simulink model "Combined_Experiment_Jan23_2020a_NoArm"  (R2020a)
settings: Solver=FixedStepAuto  StartTime=0.0  StopTime=tsim  FixedStep=baseRate  RelTol=1e-3  EnableMultiTasking=on
undefined symbols (not defined in the file): b0, b1, b_out, baseRate, CHASER_ABSOLUTE_POSITION, DiscIntNeverNeededParam, drop_states_ARM, drop_states_BLACK, drop_states_BLUE, drop_states_RED, F_Black_X_nominal, F_Black_Y_nominal, F_Blue_X_nominal, F_Blue_Y_nominal, F_red_X_nominal, F_red_Y_nominal, F_thrusters_BLACK, F_thrusters_BLUE, F_thrusters_RED, Gamma1_el, Gamma1_sh, Gamma1_wr, Gamma2_el, Gamma2_sh, Gamma2_wr, Gamma3_el, Gamma3_sh, Gamma3_wr, Gamma4_el, Gamma4_sh, Gamma4_wr, Gamma5_el, Gamma5_sh, Gamma5_wr, Gamma6_el, Gamma6_sh, Gamma6_wr, HOLD_POINT_RADIUS, home_states_BLACK, home_states_BLUE, home_states_RED, init_states_BLACK, init_states_BLUE, init_states_RED, Kd_tb, Kd_tblue, Kd_tr, Kd_xb, Kd_xblue, Kd_xr, Kd_yb, Kd_yblue, Kd_yr, Kp_tb, Kp_tblue, Kp_tr, Kp_xb, Kp_xblue, Kp_xr, Kp_yb ... (+31)
libraries: dspstat3 x18, raspberrypiBasiclib x10, dspsigops x9, embdlinuxlib x7, MainLibrary x7, simulink x7, mspfiltlib x3, dsparch4 x3, etargetslib x1, sensehatlib x1
(part 9 of 10)

== system Combined_Experiment_Jan23_2020a_NoArm/Phase #3: Experiment/Change BLACK Behavior/Sub-Phase #3 /Custom Discrete PD (Attitude)/x_dot -> x1/Hold this value ==
  In1 : Inport
  Action Port : ActionPort  ActionPortLabel=if(u1 ~= 0)
  Out1 : Outport  VectorParamsAs1DForOutWhenUnconnected=off
  wires:
  In1/1 -> Out1/1

== system Combined_Experiment_Jan23_2020a_NoArm/Phase #3: Experiment/Change BLACK Behavior/Sub-Phase #3 /Custom Discrete PD (X-Position)/x_dot -> x1/Hold this value ==
  In1 : Inport
  Action Port : ActionPort  ActionPortLabel=if(u1 ~= 0)
  Out1 : Outport  VectorParamsAs1DForOutWhenUnconnected=off
  wires:
  In1/1 -> Out1/1

== system Combined_Experiment_Jan23_2020a_NoArm/Phase #3: Experiment/Change BLACK Behavior/Sub-Phase #3 /Custom Discrete PD (Y-Position)/x_dot -> x1/Hold this value ==
  In1 : Inport
  Action Port : ActionPort  ActionPortLabel=if(u1 ~= 0)
  Out1 : Outport  VectorParamsAs1DForOutWhenUnconnected=off
  wires:
  In1/1 -> Out1/1

== system Combined_Experiment_Jan23_2020a_NoArm/Phase #3: Experiment/Change BLACK Behavior/Sub-Phase #4/Custom Discrete PD (Attitude)/x_dot -> x1/Hold this value ==
  In1 : Inport
  Action Port : ActionPort  ActionPortLabel=if(u1 ~= 0)
  Out1 : Outport  VectorParamsAs1DForOutWhenUnconnected=off
  wires:
  In1/1 -> Out1/1

== system Combined_Experiment_Jan23_2020a_NoArm/Phase #3: Experiment/Change BLACK Behavior/Sub-Phase #4/Custom Discrete PD (X-Position)/x_dot -> x1/Hold this value ==
  In1 : Inport
  Action Port : ActionPort  ActionPortLabel=if(u1 ~= 0)
  Out1 : Outport  VectorParamsAs1DForOutWhenUnconnected=off
  wires:
  In1/1 -> Out1/1

== system Combined_Experiment_Jan23_2020a_NoArm/Phase #3: Experiment/Change BLACK Behavior/Sub-Phase #4/Custom Discrete PD (Y-Position)/x_dot -> x1/Hold this value ==
  In1 : Inport
  Action Port : ActionPort  ActionPortLabel=if(u1 ~= 0)
  Out1 : Outport  VectorParamsAs1DForOutWhenUnconnected=off
  wires:
  In1/1 -> Out1/1

== system Combined_Experiment_Jan23_2020a_NoArm/Phase #3: Experiment/Change BLUE Behavior/Sub-Phase #1/Custom Discrete PD (Attitude)/x_dot -> x1/Hold this value ==
  In1 : Inport
  Action Port : ActionPort  ActionPortLabel=if(u1 ~= 0)
  Out1 : Outport  VectorParamsAs1DForOutWhenUnconnected=off
  wires:
  In1/1 -> Out1/1

== system Combined_Experiment_Jan23_2020a_NoArm/Phase #3: Experiment/Change BLUE Behavior/Sub-Phase #1/Custom Discrete PD (X-Position)/x_dot -> x1/Hold this value ==
  In1 : Inport
  Action Port : ActionPort  ActionPortLabel=if(u1 ~= 0)
  Out1 : Outport  VectorParamsAs1DForOutWhenUnconnected=off
  wires:
  In1/1 -> Out1/1

== system Combined_Experiment_Jan23_2020a_NoArm/Phase #3: Experiment/Change BLUE Behavior/Sub-Phase #1/Custom Discrete PD (Y-Position)/x_dot -> x1/Hold this value ==
  In1 : Inport
  Action Port : ActionPort  ActionPortLabel=if(u1 ~= 0)
  Out1 : Outport  VectorParamsAs1DForOutWhenUnconnected=off
  wires:
  In1/1 -> Out1/1

== system Combined_Experiment_Jan23_2020a_NoArm/Phase #3: Experiment/Change BLUE Behavior/Sub-Phase #2 /Custom Discrete PD (Attitude)/x_dot -> x1/Hold this value ==
  In1 : Inport
  Action Port : ActionPort  ActionPortLabel=if(u1 ~= 0)
  Out1 : Outport  VectorParamsAs1DForOutWhenUnconnected=off
  wires:
  In1/1 -> Out1/1

== system Combined_Experiment_Jan23_2020a_NoArm/Phase #3: Experiment/Change BLUE Behavior/Sub-Phase #2 /Custom Discrete PD (X-Position)/x_dot -> x1/Hold this value ==
  In1 : Inport
  Action Port : ActionPort  ActionPortLabel=if(u1 ~= 0)
  Out1 : Outport  VectorParamsAs1DForOutWhenUnconnected=off
  wires:
  In1/1 -> Out1/1

== system Combined_Experiment_Jan23_2020a_NoArm/Phase #3: Experiment/Change BLUE Behavior/Sub-Phase #2 /Custom Discrete PD (Y-Position)/x_dot -> x1/Hold this value ==
  In1 : Inport
  Action Port : ActionPort  ActionPortLabel=if(u1 ~= 0)
  Out1 : Outport  VectorParamsAs1DForOutWhenUnconnected=off
  wires:
  In1/1 -> Out1/1

== system Combined_Experiment_Jan23_2020a_NoArm/Phase #3: Experiment/Change BLUE Behavior/Sub-Phase #3 /Custom Discrete PD (Attitude)/x_dot -> x1/Hold this value ==
  In1 : Inport
  Action Port : ActionPort  ActionPortLabel=if(u1 ~= 0)
  Out1 : Outport  VectorParamsAs1DForOutWhenUnconnected=off
  wires:
  In1/1 -> Out1/1

== system Combined_Experiment_Jan23_2020a_NoArm/Phase #3: Experiment/Change BLUE Behavior/Sub-Phase #3 /Custom Discrete PD (X-Position)/x_dot -> x1/Hold this value ==
  In1 : Inport
  Action Port : ActionPort  ActionPortLabel=if(u1 ~= 0)
  Out1 : Outport  VectorParamsAs1DForOutWhenUnconnected=off
  wires:
  In1/1 -> Out1/1

== system Combined_Experiment_Jan23_2020a_NoArm/Phase #3: Experiment/Change BLUE Behavior/Sub-Phase #3 /Custom Discrete PD (Y-Position)/x_dot -> x1/Hold this value ==
  In1 : Inport
  Action Port : ActionPort  ActionPortLabel=if(u1 ~= 0)
  Out1 : Outport  VectorParamsAs1DForOutWhenUnconnected=off
  wires:
  In1/1 -> Out1/1

== system Combined_Experiment_Jan23_2020a_NoArm/Phase #3: Experiment/Change BLUE Behavior/Sub-Phase #4/Custom Discrete PD (Attitude)/x_dot -> x1/Hold this value ==
  In1 : Inport
  Action Port : ActionPort  ActionPortLabel=if(u1 ~= 0)
  Out1 : Outport  VectorParamsAs1DForOutWhenUnconnected=off
  wires:
  In1/1 -> Out1/1

== system Combined_Experiment_Jan23_2020a_NoArm/Phase #3: Experiment/Change BLUE Behavior/Sub-Phase #4/Custom Discrete PD (X-Position)/x_dot -> x1/Hold this value ==
  In1 : Inport
  Action Port : ActionPort  ActionPortLabel=if(u1 ~= 0)
  Out1 : Outport  VectorParamsAs1DForOutWhenUnconnected=off
  wires:
  In1/1 -> Out1/1

== system Combined_Experiment_Jan23_2020a_NoArm/Phase #3: Experiment/Change BLUE Behavior/Sub-Phase #4/Custom Discrete PD (Y-Position)/x_dot -> x1/Hold this value ==
  In1 : Inport
  Action Port : ActionPort  ActionPortLabel=if(u1 ~= 0)
  Out1 : Outport  VectorParamsAs1DForOutWhenUnconnected=off
  wires:
  In1/1 -> Out1/1

== system Combined_Experiment_Jan23_2020a_NoArm/Simulate Plant Dynamics/RED and ARM Dynamics/RED + ARM/RED + ARM Dynamics/x_dot -> x1/Hold this value ==
  In1 : Inport
  Action Port : ActionPort  ActionPortLabel=if(u1 ~= 0)
  Out1 : Outport  VectorParamsAs1DForOutWhenUnconnected=off
  wires:
  In1/1 -> Out1/1

== system Combined_Experiment_Jan23_2020a_NoArm/Simulate Plant Dynamics/RED and ARM Dynamics/RED + ARM/RED + ARM Dynamics/x_dot -> x2/Hold this value ==
  In1 : Inport
  Action Port : ActionPort  ActionPortLabel=if(u1 ~= 0)
  Out1 : Outport  VectorParamsAs1DForOutWhenUnconnected=off
  wires:
  In1/1 -> Out1/1

== system Combined_Experiment_Jan23_2020a_NoArm/Simulate Plant Dynamics/RED and ARM Dynamics/RED Only/RED Dynamics/x_dot -> x1/Hold this value ==
  In1 : Inport
  Action Port : ActionPort  ActionPortLabel=if(u1 ~= 0)
  Out1 : Outport  VectorParamsAs1DForOutWhenUnconnected=off
  wires:
  In1/1 -> Out1/1

== system Combined_Experiment_Jan23_2020a_NoArm/Simulate Plant Dynamics/RED and ARM Dynamics/RED Only/RED Dynamics/x_dot -> x2/Hold this value ==
  In1 : Inport
  Action Port : ActionPort  ActionPortLabel=if(u1 ~= 0)
  Out1 : Outport  VectorParamsAs1DForOutWhenUnconnected=off
  wires:
  In1/1 -> Out1/1

== system Combined_Experiment_Jan23_2020a_NoArm/Simulate Plant Dynamics/RED and ARM Dynamics/RED Only/RED Dynamics/x_dot -> x3/Hold this value ==
  In1 : Inport
  Action Port : ActionPort  ActionPortLabel=if(u1 ~= 0)
  Out1 : Outport  VectorParamsAs1DForOutWhenUnconnected=off
  wires:
  In1/1 -> Out1/1

== system Combined_Experiment_Jan23_2020a_NoArm/Simulate Plant Dynamics/RED and ARM Dynamics/RED Only/RED Dynamics/x_dot -> x4/Hold this value ==
  In1 : Inport
  Action Port : ActionPort  ActionPortLabel=if(u1 ~= 0)
  Out1 : Outport  VectorParamsAs1DForOutWhenUnconnected=off
  wires:
  In1/1 -> Out1/1

== system Combined_Experiment_Jan23_2020a_NoArm/Simulate Plant Dynamics/RED and ARM Dynamics/RED Only/RED Dynamics/x_dot -> x5/Hold this value ==
  In1 : Inport
  Action Port : ActionPort  ActionPortLabel=if(u1 ~= 0)
  Out1 : Outport  VectorParamsAs1DForOutWhenUnconnected=off
  wires:
  In1/1 -> Out1/1

== matlab function Combined_Experiment_Jan23_2020a_NoArm/From Force//Torque to PWM Signal/Change BLUE Behavior/Calculate Thruster ON//OFF/Rotate Forces to Inertial/Create Rotation Matrix ==
  data: Rz input; C_Ib output
function C_Ib = RotateFrame(Rz)

C_bI = [  cos(Rz) sin(Rz)
         -sin(Rz) cos(Rz) ];

C_Ib = inv(C_bI);

end

== matlab function Combined_Experiment_Jan23_2020a_NoArm/From Force//Torque to PWM Signal/Change BLUE Behavior/Rotate Forces to Body/Create Rotation Matrix ==
  data: Rz input; C_bI output
function C_bI = RotateFrame(Rz)

C_bI = [  cos(Rz) sin(Rz)
         -sin(Rz) cos(Rz) ];

end

== matlab function Combined_Experiment_Jan23_2020a_NoArm/Phase #2: Move to Initial Position/Change BLACK Behavior/Hough Control/MATLAB Function2 ==
  data: Oy output; z input; Ox output
function [Oy, Ox]   = C3( z )
%C3 gives the rotation matrix about the z-axis for an angle 'z'
%   z - the angle about the z-axis which you rotate
%   A - the rotation matrix

Ox = [cos(z) sin(z); -sin(z) cos(z)]*[1;0];
Oy = [cos(z) sin(z); -sin(z) cos(z)]*[0;1];
end

== matlab function Combined_Experiment_Jan23_2020a_NoArm/Phase #2: Move to Initial Position/Change BLACK Behavior/Hough Control/MATLAB Function3 ==
  data: z input; Ox output
function Ox    = C3( z )
%C3 gives the rotation matrix about the z-axis for an angle 'z'
%   z - the angle about the z-axis which you rotate
%   A - the rotation matrix

Ox = [cos(z) sin(z); -sin(z) cos(z)]*[1;0];
end

== matlab function Combined_Experiment_Jan23_2020a_NoArm/Phase #2: Move to Initial Position/Change BLACK Behavior/Hough Control/MATLAB Function4 ==
  data: Oy input; e_out output; e_in input
function e_out = fcn(Oy, e_in)

a = sign(Oy'*e_in);
e_out = -a*norm(e_in);

== matlab function Combined_Experiment_Jan23_2020a_NoArm/From Force//Torque to PWM Signal/Change BLACK Behavior/Calculate Thruster ON//OFF/MATLAB Function ==
  data: H output; thruster_dist2CG_BLACK parameter; F_thrusters_BLACK parameter
function H = MakeH(thruster_dist2CG_BLACK,F_thrusters_BLACK)

Vec1 = [ -1
         -1
          0 
          0
          1
          1
          0
          0 ];
      
Vec2 = [  0
          0
          1
          1
          0
          0
         -1
         -1 ];
     
Vec3 = thruster_dist2CG_BLACK./1000;

Mat1 = [Vec1, Vec2, Vec3]';

Mat2 = diag((F_thrusters_BLACK./2));

H    = Mat1*Mat2;

end

== matlab function Combined_Experiment_Jan23_2020a_NoArm/Phase #3: Experiment/Change BLACK Behavior/Sub-Phase #4/BLACK_RzD/Wrap1/MATLAB Function ==
  data: u input; wrappedAngle output
function wrappedAngle = wrapAngle(u)

wrappedAngle = atan2(sin(u),cos(u));

end

== matlab function Combined_Experiment_Jan23_2020a_NoArm/Phase #3: Experiment/Change BLACK Behavior/Sub-Phase #2 /BLACK_RzD1/Wrap1/MATLAB Function ==
  data: u input; wrappedAngle output
function wrappedAngle = wrapAngle(u)

wrappedAngle = atan2(sin(u),cos(u));

end

== matlab function Combined_Experiment_Jan23_2020a_NoArm/From Force//Torque to PWM Signal/Change BLACK Behavior/Calculate Thruster ON//OFF/MATLAB Function1 ==
  data: H output; thruster_dist2CG_BLACK parameter; F_thrusters_BLACK parameter
function H = MakeH(thruster_dist2CG_BLACK,F_thrusters_BLACK)

Vec1 = [ -1
         -1
          0 
          0
          1
          1
          0
          0 ];
      
Vec2 = [  0
          0
          1
          1
          0
          0
         -1
         -1 ];
     
Vec3 = thruster_dist2CG_BLACK./1000;

Mat1 = [Vec1, Vec2, Vec3]';

Mat2 = diag((F_thrusters_BLACK));

H    = Mat1*Mat2;

end

== matlab function Combined_Experiment_Jan23_2020a_NoArm/From Force//Torque to PWM Signal/Change BLACK Behavior/Calculate Thruster ON//OFF/MATLAB Function2 ==
  data: ThrustPer_Final output; ThrustPer input
function ThrustPer_Final  = ThrusterSat(ThrustPer)

ValveTime       = 0.007;
TControl        = 0.1;
ThrustPer_Final = zeros(8,1);

if max(ThrustPer) > 1
    ThrustPer_Sat = ThrustPer/max(ThrustPer);
else
    ThrustPer_Sat = ThrustPer;
end

for i = 1:8
    if ThrustPer_Sat(i) > ValveTime/TControl 
        ThrustPer_Final(i) = ThrustPer_Sat(i);
    else
        ThrustPer_Final(i) = 0;
    end
end
   

end

== matlab function Combined_Experiment_Jan23_2020a_NoArm/From Force//Torque to PWM Signal/Change BLACK Behavior/Calculate Thruster ON//OFF/Rotate Forces to Inertial/Create Rotation Matrix ==
  data: Rz input; C_Ib output
function C_Ib = RotateFrame(Rz)

C_bI = [  cos(Rz) sin(Rz)
         -sin(Rz) cos(Rz) ];

C_Ib = inv(C_bI);

end

== matlab function Combined_Experiment_Jan23_2020a_NoArm/From Force//Torque to PWM Signal/Change BLACK Behavior/Rotate Forces to Body/Create Rotation Matrix ==
  data: Rz input; C_bI output
function C_bI = RotateFrame(Rz)

C_bI = [  cos(Rz) sin(Rz)
         -sin(Rz) cos(Rz) ];

end

== matlab function Combined_Experiment_Jan23_2020a_NoArm/Phase #3: Experiment/Change RED Behavior/Sub-Phase #2 /calculate_mass_matrix ==
  data: M output
function M  = generate_M()
  
    m0                 = 11.211000;     % RED Mass
    I0                = 0.202150;      % RED Inertia;
    
    m1               = 0.345;       % ARM m1
    m2                = 0.335;       % ARM m2
    m3                = 0.111;       % ARM m3


    M = [m0+m1+m2+m3 0 0
         0 m0+m1+m2+m3 0
         0 0 I0];

end
% Artificially setting M_31 and M_32 to zero, such that the feedforward
% controller does not think a torque needs to be applied to the base to
% counteract the torque needed to maintain the angular acceleration of the
% links when the base has a linear acceleration. No torque is applied to keep the links at their linear
% acceleration because friction does this for us.

% The original matrix
% M = reshape([t17,0.0,t30,-t86-t87-t88,-t88-t13.*t28,-t88,...
%     0.0,t17,t33,-t89-t90-t91,-t91-t24.*t28,-t91,...
%     t30,t33,...
%     I0+I1+I2+I3+t46+t51+t57+t64+t65+t66+t67+t68+t70+t71+t72+t74+t75+t76+t77+t59.*(a1.*b0.*m1.*2.0+a1.*b0.*m2.*2.0+a1.*b0.*m3.*2.0+b0.*b1.*m2.*2.0+b0.*b1.*m3.*2.0)+m1.*t36+m2.*t36+m3.*t36-t61.*(a2.*b0.*m2.*2.0+a2.*b0.*m3.*2.0+b0.*b2.*m3.*2.0)-a3.*b0.*m3.*t63.*2.0,t99,I2+I3+t51+t67+t68+t70+t74+t77+t85+t107-t112-t113,I3+t70+t85+t111-t113,-t7.*t8-t13.*t14-a3.*m3.*t16,    -t8.*t23-t14.*t24-a3.*m3.*t25,t99,I1+I2+I3+t46+t51+t57+t64+t65+t66+t67+t68+t70+t71+t72+t74+t75+t76+t77,t114,t115,-t13.*t28-a3.*m3.*t16,-t24.*t28-a3.*m3.*t25,I2+I3+t51+t67+t68+t70+t74+t77+t85+t107-t61.*t81-a3.*b0.*m3.*t63,t114,I2+I3+t51+t67+t68+t70+t74+t77,t116,-a3.*m3.*t16,-a3.*m3.*t25,I3+t70+t85+t111-a3.*b0.*m3.*t63,t115,t116,I3+t70],[6,6]);

== matlab function Combined_Experiment_Jan23_2020a_NoArm/Phase #3: Experiment/Change RED Behavior/Sub-Phase #3 /calculate_mass_matrix ==
  data: M output
function M  = generate_M()
  
    m0                 = 11.211000;     % RED Mass
    I0                = 0.202150;      % RED Inertia;
    
    m1               = 0.345;       % ARM m1
    m2                = 0.335;       % ARM m2
    m3                = 0.111;       % ARM m3


    M = [m0+m1+m2+m3 0 0
         0 m0+m1+m2+m3 0
         0 0 I0];

end
% Artificially setting M_31 and M_32 to zero, such that the feedforward
% controller does not think a torque needs to be applied to the base to
% counteract the torque needed to maintain the angular acceleration of the
% links when the base has a linear acceleration. No torque is applied to keep the links at their linear
% acceleration because friction does this for us.

% The original matrix
% M = reshape([t17,0.0,t30,-t86-t87-t88,-t88-t13.*t28,-t88,...
%     0.0,t17,t33,-t89-t90-t91,-t91-t24.*t28,-t91,...
%     t30,t33,...
%     I0+I1+I2+I3+t46+t51+t57+t64+t65+t66+t67+t68+t70+t71+t72+t74+t75+t76+t77+t59.*(a1.*b0.*m1.*2.0+a1.*b0.*m2.*2.0+a1.*b0.*m3.*2.0+b0.*b1.*m2.*2.0+b0.*b1.*m3.*2.0)+m1.*t36+m2.*t36+m3.*t36-t61.*(a2.*b0.*m2.*2.0+a2.*b0.*m3.*2.0+b0.*b2.*m3.*2.0)-a3.*b0.*m3.*t63.*2.0,t99,I2+I3+t51+t67+t68+t70+t74+t77+t85+t107-t112-t113,I3+t70+t85+t111-t113,-t7.*t8-t13.*t14-a3.*m3.*t16,    -t8.*t23-t14.*t24-a3.*m3.*t25,t99,I1+I2+I3+t46+t51+t57+t64+t65+t66+t67+t68+t70+t71+t72+t74+t75+t76+t77,t114,t115,-t13.*t28-a3.*m3.*t16,-t24.*t28-a3.*m3.*t25,I2+I3+t51+t67+t68+t70+t74+t77+t85+t107-t61.*t81-a3.*b0.*m3.*t63,t114,I2+I3+t51+t67+t68+t70+t74+t77,t116,-a3.*m3.*t16,-a3.*m3.*t25,I3+t70+t85+t111-a3.*b0.*m3.*t63,t115,t116,I3+t70],[6,6]);

== matlab function Combined_Experiment_Jan23_2020a_NoArm/Phase #3: Experiment/Change RED Behavior/Sub-Phase #4/calculate_mass_matrix ==
  data: M output
function M  = generate_M()
  
    m0                 = 11.211000;     % RED Mass
    I0                = 0.202150;      % RED Inertia;
    
    m1               = 0.345;       % ARM m1
    m2                = 0.335;       % ARM m2
    m3                = 0.111;       % ARM m3


    M = [m0+m1+m2+m3 0 0
         0 m0+m1+m2+m3 0
         0 0 I0];

end
% Artificially setting M_31 and M_32 to zero, such that the feedforward
% controller does not think a torque needs to be applied to the base to
% counteract the torque needed to maintain the angular acceleration of the
% links when the base has a linear acceleration. No torque is applied to keep the links at their linear
% acceleration because friction does this for us.

% The original matrix
% M = reshape([t17,0.0,t30,-t86-t87-t88,-t88-t13.*t28,-t88,...
%     0.0,t17,t33,-t89-t90-t91,-t91-t24.*t28,-t91,...
%     t30,t33,...
%     I0+I1+I2+I3+t46+t51+t57+t64+t65+t66+t67+t68+t70+t71+t72+t74+t75+t76+t77+t59.*(a1.*b0.*m1.*2.0+a1.*b0.*m2.*2.0+a1.*b0.*m3.*2.0+b0.*b1.*m2.*2.0+b0.*b1.*m3.*2.0)+m1.*t36+m2.*t36+m3.*t36-t61.*(a2.*b0.*m2.*2.0+a2.*b0.*m3.*2.0+b0.*b2.*m3.*2.0)-a3.*b0.*m3.*t63.*2.0,t99,I2+I3+t51+t67+t68+t70+t74+t77+t85+t107-t112-t113,I3+t70+t85+t111-t113,-t7.*t8-t13.*t14-a3.*m3.*t16,    -t8.*t23-t14.*t24-a3.*m3.*t25,t99,I1+I2+I3+t46+t51+t57+t64+t65+t66+t67+t68+t70+t71+t72+t74+t75+t76+t77,t114,t115,-t13.*t28-a3.*m3.*t16,-t24.*t28-a3.*m3.*t25,I2+I3+t51+t67+t68+t70+t74+t77+t85+t107-t61.*t81-a3.*b0.*m3.*t63,t114,I2+I3+t51+t67+t68+t70+t74+t77,t116,-a3.*m3.*t16,-a3.*m3.*t25,I3+t70+t85+t111-a3.*b0.*m3.*t63,t115,t116,I3+t70],[6,6]);

== matlab function Combined_Experiment_Jan23_2020a_NoArm/Simulate Plant Dynamics/RED and ARM Dynamics/RED Only/RED Dynamics/Sample and Hold Data to Match PhaseSpace (RED)/MATLAB Function ==
  data: TIME input; y output; SERVER input
function y = fcn(TIME, SERVER)

if mod(TIME,SERVER) == 0
    y = 1;
else
    y = 0;
end

== matlab function Combined_Experiment_Jan23_2020a_NoArm/Simulate Plant Dynamics/BLACK Dynamics/Sample and Hold Data to Match PhaseSpace (BLACK)/MATLAB Function ==
  data: TIME input; y output; SERVER input
function y = fcn(TIME, SERVER)

if mod(TIME,SERVER) == 0
    y = 1;
else
    y = 0;
end

== matlab function Combined_Experiment_Jan23_2020a_NoArm/From Force//Torque to PWM Signal/Change RED Behavior/Rotate Forces to Body/Create Rotation Matrix ==
  data: Rz input; C_bI output
function C_bI = RotateFrame(Rz)

C_bI = [  cos(Rz) sin(Rz)
         -sin(Rz) cos(Rz) ];

end

== matlab function Combined_Experiment_Jan23_2020a_NoArm/Phase #2: Move to Initial Position/Change RED Behavior/Hough Control/MATLAB Function2 ==
  data: Oy output; z input; Ox output
function [Oy, Ox]   = C3( z )
%C3 gives the rotation matrix about the z-axis for an angle 'z'
%   z - the angle about the z-axis which you rotate
%   A - the rotation matrix

Ox = [cos(z) sin(z); -sin(z) cos(z)]*[1;0];
Oy = [cos(z) sin(z); -sin(z) cos(z)]*[0;1];
end

== matlab function Combined_Experiment_Jan23_2020a_NoArm/Phase #2: Move to Initial Position/Change RED Behavior/Hough Control/MATLAB Function3 ==
  data: z input; Ox output
function Ox    = C3( z )
%C3 gives the rotation matrix about the z-axis for an angle 'z'
%   z - the angle about the z-axis which you rotate
%   A - the rotation matrix

Ox = [cos(z) sin(z); -sin(z) cos(z)]*[1;0];
end

== matlab function Combined_Experiment_Jan23_2020a_NoArm/Phase #2: Move to Initial Position/Change RED Behavior/Hough Control/MATLAB Function4 ==
  data: Oy input; e_out output; e_in input
function e_out = fcn(Oy, e_in)

a = sign(Oy'*e_in);
e_out = -a*norm(e_in);

== matlab function Combined_Experiment_Jan23_2020a_NoArm/Phase #3: Experiment/Change BLACK Behavior/Sub-Phase #2 /Hough Control/MATLAB Function2 ==
  data: Oy output; z input; Ox output
function [Oy, Ox]   = C3( z )
%C3 gives the rotation matrix about the z-axis for an angle 'z'
%   z - the angle about the z-axis which you rotate
%   A - the rotation matrix

Ox = [cos(z) sin(z); -sin(z) cos(z)]*[1;0];
Oy = [cos(z) sin(z); -sin(z) cos(z)]*[0;1];
end

== matlab function Combined_Experiment_Jan23_2020a_NoArm/Phase #4: Return Home/Change BLACK Behavior/Hough Control/MATLAB Function2 ==
  data: Oy output; z input; Ox output
function [Oy, Ox]   = C3( z )
%C3 gives the rotation matrix about the z-axis for an angle 'z'
%   z - the angle about the z-axis which you rotate
%   A - the rotation matrix

Ox = [cos(z) sin(z); -sin(z) cos(z)]*[1;0];
Oy = [cos(z) sin(z); -sin(z) cos(z)]*[0;1];
end

== matlab function Combined_Experiment_Jan23_2020a_NoArm/Phase #4: Return Home/Change BLACK Behavior/Hough Control/MATLAB Function3 ==
  data: z input; Ox output
function Ox    = C3( z )
%C3 gives the rotation matrix about the z-axis for an angle 'z'
%   z - the angle about the z-axis which you rotate
%   A - the rotation matrix

Ox = [cos(z) sin(z); -sin(z) cos(z)]*[1;0];
end

== matlab function Combined_Experiment_Jan23_2020a_NoArm/Phase #4: Return Home/Change BLACK Behavior/Hough Control/MATLAB Function4 ==
  data: Oy input; e_out output; e_in input
function e_out = fcn(Oy, e_in)

a = sign(Oy'*e_in);
e_out = -a*norm(e_in);

== matlab function Combined_Experiment_Jan23_2020a_NoArm/Phase #4: Return Home/Change RED Behavior/Hough Control/MATLAB Function2 ==
  data: Oy output; z input; Ox output
function [Oy, Ox]   = C3( z )
%C3 gives the rotation matrix about the z-axis for an angle 'z'
%   z - the angle about the z-axis which you rotate
%   A - the rotation matrix

Ox = [cos(z) sin(z); -sin(z) cos(z)]*[1;0];
Oy = [cos(z) sin(z); -sin(z) cos(z)]*[0;1];
end

== matlab function Combined_Experiment_Jan23_2020a_NoArm/Phase #4: Return Home/Change RED Behavior/Hough Control/MATLAB Function3 ==
  data: z input; Ox output
function Ox    = C3( z )
%C3 gives the rotation matrix about the z-axis for an angle 'z'
%   z - the angle about the z-axis which you rotate
%   A - the rotation matrix

Ox = [cos(z) sin(z); -sin(z) cos(z)]*[1;0];
end

== matlab function Combined_Experiment_Jan23_2020a_NoArm/Phase #4: Return Home/Change RED Behavior/Hough Control/MATLAB Function4 ==
  data: Oy input; e_out output; e_in input
function e_out = fcn(Oy, e_in)

a = sign(Oy'*e_in);
e_out = -a*norm(e_in);

== matlab function Combined_Experiment_Jan23_2020a_NoArm/Phase #2: Move to Initial Position/Change BLUE Behavior/Hough Control/MATLAB Function2 ==
  data: Oy output; z input; Ox output
function [Oy, Ox]   = C3( z )
%C3 gives the rotation matrix about the z-axis for an angle 'z'
%   z - the angle about the z-axis which you rotate
%   A - the rotation matrix

Ox = [cos(z) sin(z); -sin(z) cos(z)]*[1;0];
Oy = [cos(z) sin(z); -sin(z) cos(z)]*[0;1];
end

== matlab function Combined_Experiment_Jan23_2020a_NoArm/Phase #2: Move to Initial Position/Change BLUE Behavior/Hough Control/MATLAB Function3 ==
  data: z input; Ox output
function Ox    = C3( z )
%C3 gives the rotation matrix about the z-axis for an angle 'z'
%   z - the angle about the z-axis which you rotate
%   A - the rotation matrix

Ox = [cos(z) sin(z); -sin(z) cos(z)]*[1;0];
end

== matlab function Combined_Experiment_Jan23_2020a_NoArm/Phase #2: Move to Initial Position/Change BLUE Behavior/Hough Control/MATLAB Function4 ==
  data: Oy input; e_out output; e_in input
function e_out = fcn(Oy, e_in)

a = sign(Oy'*e_in);
e_out = -a*norm(e_in);

== matlab function Combined_Experiment_Jan23_2020a_NoArm/Phase #3: Experiment/Change BLUE Behavior/Sub-Phase #1/BLACK_RzD1/Wrap1/MATLAB Function ==
  data: u input; wrappedAngle output
function wrappedAngle = wrapAngle(u)

wrappedAngle = atan2(sin(u),cos(u));

end

== matlab function Combined_Experiment_Jan23_2020a_NoArm/Phase #3: Experiment/Change BLACK Behavior/Sub-Phase #2 /Hough Control/MATLAB Function3 ==
  data: z input; Ox output
function Ox    = C3( z )
%C3 gives the rotation matrix about the z-axis for an angle 'z'
%   z - the angle about the z-axis which you rotate
%   A - the rotation matrix

Ox = [cos(z) sin(z); -sin(z) cos(z)]*[1;0];
end

== matlab function Combined_Experiment_Jan23_2020a_NoArm/Phase #3: Experiment/Change RED Behavior/Sub-Phase #1/calculate_mass_matrix ==
  data: M output
function M  = generate_M()
  
    m0                 = 11.211000;     % RED Mass
    I0                = 0.202150;      % RED Inertia;
    
    m1               = 0.345;       % ARM m1
    m2                = 0.335;       % ARM m2
    m3                = 0.111;       % ARM m3


    M = [m0+m1+m2+m3 0 0
         0 m0+m1+m2+m3 0
         0 0 I0];

end
% Artificially setting M_31 and M_32 to zero, such that the feedforward
% controller does not think a torque needs to be applied to the base to
% counteract the torque needed to maintain the angular acceleration of the
% links when the base has a linear acceleration. No torque is applied to keep the links at their linear
% acceleration because friction does this for us.

% The original matrix
% M = reshape([t17,0.0,t30,-t86-t87-t88,-t88-t13.*t28,-t88,...
%     0.0,t17,t33,-t89-t90-t91,-t91-t24.*t28,-t91,...
%     t30,t33,...
%     I0+I1+I2+I3+t46+t51+t57+t64+t65+t66+t67+t68+t70+t71+t72+t74+t75+t76+t77+t59.*(a1.*b0.*m1.*2.0+a1.*b0.*m2.*2.0+a1.*b0.*m3.*2.0+b0.*b1.*m2.*2.0+b0.*b1.*m3.*2.0)+m1.*t36+m2.*t36+m3.*t36-t61.*(a2.*b0.*m2.*2.0+a2.*b0.*m3.*2.0+b0.*b2.*m3.*2.0)-a3.*b0.*m3.*t63.*2.0,t99,I2+I3+t51+t67+t68+t70+t74+t77+t85+t107-t112-t113,I3+t70+t85+t111-t113,-t7.*t8-t13.*t14-a3.*m3.*t16,    -t8.*t23-t14.*t24-a3.*m3.*t25,t99,I1+I2+I3+t46+t51+t57+t64+t65+t66+t67+t68+t70+t71+t72+t74+t75+t76+t77,t114,t115,-t13.*t28-a3.*m3.*t16,-t24.*t28-a3.*m3.*t25,I2+I3+t51+t67+t68+t70+t74+t77+t85+t107-t61.*t81-a3.*b0.*m3.*t63,t114,I2+I3+t51+t67+t68+t70+t74+t77,t116,-a3.*m3.*t16,-a3.*m3.*t25,I3+t70+t85+t111-a3.*b0.*m3.*t63,t115,t116,I3+t70],[6,6]);

== matlab function Combined_Experiment_Jan23_2020a_NoArm/Phase #3: Experiment/Change BLACK Behavior/Sub-Phase #2 /Hough Control/MATLAB Function4 ==
  data: Oy input; e_out output; e_in input
function e_out = fcn(Oy, e_in)

a = sign(Oy'*e_in);
e_out = -a*norm(e_in);

== matlab function Combined_Experiment_Jan23_2020a_NoArm/Phase #3: Experiment/Change BLUE Behavior/Sub-Phase #1/Hough Control/MATLAB Function2 ==
  data: Oy output; z input; Ox output
function [Oy, Ox]   = C3( z )
%C3 gives the rotation matrix about the z-axis for an angle 'z'
%   z - the angle about the z-axis which you rotate
%   A - the rotation matrix

Ox = [cos(z) sin(z); -sin(z) cos(z)]*[1;0];
Oy = [cos(z) sin(z); -sin(z) cos(z)]*[0;1];
end

== matlab function Combined_Experiment_Jan23_2020a_NoArm/Phase #3: Experiment/Change BLUE Behavior/Sub-Phase #1/Hough Control/MATLAB Function3 ==
  data: z input; Ox output
function Ox    = C3( z )
%C3 gives the rotation matrix about the z-axis for an angle 'z'
%   z - the angle about the z-axis which you rotate
%   A - the rotation matrix

Ox = [cos(z) sin(z); -sin(z) cos(z)]*[1;0];
end

== matlab function Combined_Experiment_Jan23_2020a_NoArm/Phase #3: Experiment/Change BLUE Behavior/Sub-Phase #4/BLACK_RzD1/Wrap1/MATLAB Function ==
  data: u input; wrappedAngle output
function wrappedAngle = wrapAngle(u)

wrappedAngle = atan2(sin(u),cos(u));

end

== matlab function Combined_Experiment_Jan23_2020a_NoArm/Phase #3: Experiment/Change BLACK Behavior/Sub-Phase #3 /BLACK_RzD1/Wrap1/MATLAB Function ==
  data: u input; wrappedAngle output
function wrappedAngle = wrapAngle(u)

wrappedAngle = atan2(sin(u),cos(u));

end

== matlab function Combined_Experiment_Jan23_2020a_NoArm/Jetson Communication/Kirk Network Control (SIM)/MATLAB Function ==
  data: Pi_time input; Ax_command output; Pi_red_x input; Pi_red_y input; Pi_red_theta input; Pi_red_Vx input; Pi_red_Vy input; Pi_red_omega input; Pi_black_x input; Pi_black_y input; Pi_black_theta input; Pi_black_Vx input; Pi_black_Vy input; Pi_black_omega input; Ay_command output; Az_command output; CHASER_ABSOLUTE_POSITION parameter; HOLD_POINT_RADIUS parameter; relevant_state_mean parameter; relevant_half_range parameter; w0 parameter; b0 parameter; w1 parameter; b1 parameter; w_out parameter; b_out parameter; MAX_VELOCITY parameter; MAX_BODY_ANGULAR_VELOCITY parameter
function [Ax_command, Ay_command, Az_command] = guidance_server_sim(Pi_time, Pi_red_x, Pi_red_y, Pi_red_theta, Pi_red_Vx, Pi_red_Vy,...
                                 Pi_red_omega, Pi_black_x, Pi_black_y, Pi_black_theta, Pi_black_Vx,...
                                 Pi_black_Vy, Pi_black_omega, CHASER_ABSOLUTE_POSITION, HOLD_POINT_RADIUS,...
                                 relevant_state_mean, relevant_half_range, w0, b0, w1, b1, w_out, b_out, MAX_VELOCITY,...
                                 MAX_BODY_ANGULAR_VELOCITY)
    % For testing
    SPOTNet_sees_target = false;
    VELOCITY_LIMIT = [MAX_VELOCITY, MAX_VELOCITY,MAX_BODY_ANGULAR_VELOCITY]; 
    
    
    if SPOTNet_sees_target == true
        
        % Insert logic that uses the vision data
        
        output = [0,0,0];
        
    else
        
        % We don't see the target -> Use PhaseSpace only
        % Calculating the relative X and Y in the chaser's body frame using PhaseSpace
        relative_pose_inertial = [Pi_black_x - Pi_red_x, Pi_black_y - Pi_red_y, Pi_black_theta - Pi_red_theta];
        
        % Calculate the roation matrix from inertia to body
        C_bI_red = [ cos(Pi_red_theta), sin(Pi_red_theta);...
                -sin(Pi_red_theta), cos(Pi_red_theta)];
        
        % Calculate relative body pose    
        %relative_pose_body     = C_bI_red*relative_pose_inertial;
        
        % With chaser absolute position
        % policy_input = np.array([relative_pose_body[0] - self.offset_x, relative_pose_body[1] - self.offset_y, (self.SPOTNet_target_angle_inertial - Pi_red_theta - self.offset_angle)%(2*np.pi), Pi_red_x, Pi_red_y, Pi_red_theta, Pi_red_Vx, Pi_red_Vy, Pi_red_omega, Pi_black_omega])

        %############# New policy input as of Nov 9 2022                    
        % Calculate the desired X, Y, theta, Vx, Vy, omega 
        % relative to the chaser's current state
        % all in the inertial frame                 

        %Calculate desired position and velocity in the inertial frame
        desired_position_relative_to_target_I = [-sin(Pi_black_theta)*(HOLD_POINT_RADIUS), cos(Pi_black_theta)*(HOLD_POINT_RADIUS), -pi/2];
        desired_position_I = [Pi_black_x, Pi_black_y, Pi_black_theta] + desired_position_relative_to_target_I;
        desired_velocity_I = [Pi_black_Vx, Pi_black_Vy, Pi_black_omega] + cross([0,0,Pi_black_omega], desired_position_relative_to_target_I);

        % Now calculate the chaser's relative position and velocity to that desired location and velocity in the inertial frame
        chaser_position_error_inertial = desired_position_I - [Pi_red_x, Pi_red_y, Pi_red_theta];
        chaser_velocity_error_inertial = desired_velocity_I - [Pi_red_Vx, Pi_red_Vy, Pi_red_omega];
        policy_input = [Pi_red_x, Pi_red_y, mod(Pi_red_theta, 2*pi), Pi_red_Vx, Pi_red_Vy, Pi_red_omega, relative_pose_inertial, chaser_position_error_inertial, chaser_velocity_error_inertial];

        % Normalize the states
        normalized_policy_input = (policy_input - relevant_state_mean)./relevant_half_range;
        
        % Run the policy input through the neural network
        
        % First fully-connected layer
        layer_1 = max(0,normalized_policy_input*w0 + b0);

        % Second fully-connected layer
        layer_2 = max(0,layer_1*w1 + b1);

        % Output layer
        output = tanh(layer_2*w_out + b_out);
        
        % Convert commands
        output(1) = output(1).*0.02;
        output(2) = output(2).*0.02;
        output(3) = output(3).*0.05;
        
        % Transform back to inertial
        %output(1:2) = C_bI_red'*output(1:2)';
        
        % Cap the velocities if they exceed limits
        % Checking whether our velocity is too large AND the acceleration is trying to increase said velocity... in which case we set the desired_linear_acceleration to zero.
    	% this is in the inertial frame							   
        current_velocity = [Pi_red_Vx, Pi_red_Vy, Pi_red_omega];
        
        if abs(current_velocity(1)) > VELOCITY_LIMIT(1) && sign(output(1))==sign(current_velocity(1))
            
            output(1) = 0;
            
        end
        
        if abs(current_velocity(2)) > VELOCITY_LIMIT(2) && sign(output(2))==sign(current_velocity(2))
            
            output(2) = 0;
            
        end
        
        if abs(current_velocity(3)) > VELOCITY_LIMIT(3) && sign(output(3))==sign(current_velocity(3))
            
            output(3) = 0;
            
        end
        
    end
    
    Ax_command = output(1);
    Ay_command = output(2);
    Az_command = output(3);
                             
end

== matlab function Combined_Experiment_Jan23_2020a_NoArm/Phase #3: Experiment/Change BLACK Behavior/Sub-Phase #3 /Hough Control/MATLAB Function2 ==
  data: Oy output; z input; Ox output
function [Oy, Ox]   = C3( z )
%C3 gives the rotation matrix about the z-axis for an angle 'z'
%   z - the angle about the z-axis which you rotate
%   A - the rotation matrix

Ox = [cos(z) sin(z); -sin(z) cos(z)]*[1;0];
Oy = [cos(z) sin(z); -sin(z) cos(z)]*[0;1];
end

== matlab function Combined_Experiment_Jan23_2020a_NoArm/Phase #3: Experiment/Change BLACK Behavior/Sub-Phase #3 /Hough Control/MATLAB Function3 ==
  data: z input; Ox output
function Ox    = C3( z )
%C3 gives the rotation matrix about the z-axis for an angle 'z'
%   z - the angle about the z-axis which you rotate
%   A - the rotation matrix

Ox = [cos(z) sin(z); -sin(z) cos(z)]*[1;0];
end

== matlab function Combined_Experiment_Jan23_2020a_NoArm/Phase #3: Experiment/Change BLACK Behavior/Sub-Phase #1/BLACK_RzD1/Wrap1/MATLAB Function ==
  data: u input; wrappedAngle output
function wrappedAngle = wrapAngle(u)

wrappedAngle = atan2(sin(u),cos(u));

end

== matlab function Combined_Experiment_Jan23_2020a_NoArm/Phase #3: Experiment/Change BLACK Behavior/Sub-Phase #1/Hough Control/MATLAB Function2 ==
  data: Oy output; z input; Ox output
function [Oy, Ox]   = C3( z )
%C3 gives the rotation matrix about the z-axis for an angle 'z'
%   z - the angle about the z-axis which you rotate
%   A - the rotation matrix

Ox = [cos(z) sin(z); -sin(z) cos(z)]*[1;0];
Oy = [cos(z) sin(z); -sin(z) cos(z)]*[0;1];
end

== matlab function Combined_Experiment_Jan23_2020a_NoArm/Phase #3: Experiment/Change BLACK Behavior/Sub-Phase #1/Hough Control/MATLAB Function3 ==
  data: z input; Ox output
function Ox    = C3( z )
%C3 gives the rotation matrix about the z-axis for an angle 'z'
%   z - the angle about the z-axis which you rotate
%   A - the rotation matrix

Ox = [cos(z) sin(z); -sin(z) cos(z)]*[1;0];
end

== matlab function Combined_Experiment_Jan23_2020a_NoArm/Phase #3: Experiment/Change BLUE Behavior/Sub-Phase #4/Hough Control/MATLAB Function2 ==
  data: Oy output; z input; Ox output
function [Oy, Ox]   = C3( z )
%C3 gives the rotation matrix about the z-axis for an angle 'z'
%   z - the angle about the z-axis which you rotate
%   A - the rotation matrix

Ox = [cos(z) sin(z); -sin(z) cos(z)]*[1;0];
Oy = [cos(z) sin(z); -sin(z) cos(z)]*[0;1];
end

== matlab function Combined_Experiment_Jan23_2020a_NoArm/Phase #3: Experiment/Change BLUE Behavior/Sub-Phase #4/Hough Control/MATLAB Function3 ==
  data: z input; Ox output
function Ox    = C3( z )
%C3 gives the rotation matrix about the z-axis for an angle 'z'
%   z - the angle about the z-axis which you rotate
%   A - the rotation matrix

Ox = [cos(z) sin(z); -sin(z) cos(z)]*[1;0];
end

== matlab function Combined_Experiment_Jan23_2020a_NoArm/Phase #5: Hold Home/Change BLACK Behavior/Hough Control/MATLAB Function2 ==
  data: Oy output; z input; Ox output
function [Oy, Ox]   = C3( z )
%C3 gives the rotation matrix about the z-axis for an angle 'z'
%   z - the angle about the z-axis which you rotate
%   A - the rotation matrix

Ox = [cos(z) sin(z); -sin(z) cos(z)]*[1;0];
Oy = [cos(z) sin(z); -sin(z) cos(z)]*[0;1];
end

== matlab function Combined_Experiment_Jan23_2020a_NoArm/Simulate Plant Dynamics/BLUE Dynamics/BLUE  Dynamics Model/MATLAB Function ==
  data: control_inputs input; x_ddot output; model_param parameter
function x_ddot = BLUE_dynamics(control_inputs, model_param)

%#codegen
% Fully define the size of x_ddot() for code generation:
x_ddot     = zeros(3,1);

% Extract the servicer model parameters from the model_param vector defined
% in initialize.m:
m_BLUE    = model_param(5);
I_BLUE    = model_param(6);

% Extract the control inputs from the control_input vector:
Fx        = control_inputs(1);              % [N]
Fy        = control_inputs(2);              % [N]
Tz        = control_inputs(3);              % [N.m]

% Calculate the state acceleration vector:
x_ddot(1) = Fx/m_BLUE;                      % [m/s^2]
x_ddot(2) = Fy/m_BLUE;                      % [m/s^2]
x_ddot(3) = Tz/I_BLUE;                      % [rad/s^2]

end

== matlab function Combined_Experiment_Jan23_2020a_NoArm/Phase #5: Hold Home/Change BLACK Behavior/Hough Control/MATLAB Function3 ==
  data: z input; Ox output
function Ox    = C3( z )
%C3 gives the rotation matrix about the z-axis for an angle 'z'
%   z - the angle about the z-axis which you rotate
%   A - the rotation matrix

Ox = [cos(z) sin(z); -sin(z) cos(z)]*[1;0];
end

== matlab function Combined_Experiment_Jan23_2020a_NoArm/Phase #5: Hold Home/Change BLACK Behavior/Hough Control/MATLAB Function4 ==
  data: Oy input; e_out output; e_in input
function e_out = fcn(Oy, e_in)

a = sign(Oy'*e_in);
e_out = -a*norm(e_in);

== matlab function Combined_Experiment_Jan23_2020a_NoArm/Phase #4: Return Home/Change BLUE Behavior/Hough Control/MATLAB Function2 ==
  data: Oy output; z input; Ox output
function [Oy, Ox]   = C3( z )
%C3 gives the rotation matrix about the z-axis for an angle 'z'
%   z - the angle about the z-axis which you rotate
%   A - the rotation matrix

Ox = [cos(z) sin(z); -sin(z) cos(z)]*[1;0];
Oy = [cos(z) sin(z); -sin(z) cos(z)]*[0;1];
end

== matlab function Combined_Experiment_Jan23_2020a_NoArm/Phase #4: Return Home/Change BLUE Behavior/Hough Control/MATLAB Function3 ==
  data: z input; Ox output
function Ox    = C3( z )
%C3 gives the rotation matrix about the z-axis for an angle 'z'
%   z - the angle about the z-axis which you rotate
%   A - the rotation matrix

Ox = [cos(z) sin(z); -sin(z) cos(z)]*[1;0];
end

== matlab function Combined_Experiment_Jan23_2020a_NoArm/Phase #4: Return Home/Change BLUE Behavior/Hough Control/MATLAB Function4 ==
  data: Oy input; e_out output; e_in input
function e_out = fcn(Oy, e_in)

a = sign(Oy'*e_in);
e_out = -a*norm(e_in);

== matlab function Combined_Experiment_Jan23_2020a_NoArm/Phase #3: Experiment/Change BLUE Behavior/Sub-Phase #2 /BLACK_RzD1/Wrap1/MATLAB Function ==
  data: u input; wrappedAngle output
function wrappedAngle = wrapAngle(u)

wrappedAngle = atan2(sin(u),cos(u));

end

== matlab function Combined_Experiment_Jan23_2020a_NoArm/Phase #3: Experiment/Change BLUE Behavior/Sub-Phase #2 /Hough Control/MATLAB Function2 ==
  data: Oy output; z input; Ox output
function [Oy, Ox]   = C3( z )
%C3 gives the rotation matrix about the z-axis for an angle 'z'
%   z - the angle about the z-axis which you rotate
%   A - the rotation matrix

Ox = [cos(z) sin(z); -sin(z) cos(z)]*[1;0];
Oy = [cos(z) sin(z); -sin(z) cos(z)]*[0;1];
end

== matlab function Combined_Experiment_Jan23_2020a_NoArm/Phase #3: Experiment/Change BLUE Behavior/Sub-Phase #2 /Hough Control/MATLAB Function3 ==
  data: z input; Ox output
function Ox    = C3( z )
%C3 gives the rotation matrix about the z-axis for an angle 'z'
%   z - the angle about the z-axis which you rotate
%   A - the rotation matrix

Ox = [cos(z) sin(z); -sin(z) cos(z)]*[1;0];
end

== matlab function Combined_Experiment_Jan23_2020a_NoArm/Phase #5: Hold Home/Change BLUE Behavior/Hough Control/MATLAB Function2 ==
  data: Oy output; z input; Ox output
function [Oy, Ox]   = C3( z )
%C3 gives the rotation matrix about the z-axis for an angle 'z'
%   z - the angle about the z-axis which you rotate
%   A - the rotation matrix

Ox = [cos(z) sin(z); -sin(z) cos(z)]*[1;0];
Oy = [cos(z) sin(z); -sin(z) cos(z)]*[0;1];
end

== matlab function Combined_Experiment_Jan23_2020a_NoArm/Phase #5: Hold Home/Change BLUE Behavior/Hough Control/MATLAB Function3 ==
  data: z input; Ox output
function Ox    = C3( z )
%C3 gives the rotation matrix about the z-axis for an angle 'z'
%   z - the angle about the z-axis which you rotate
%   A - the rotation matrix

Ox = [cos(z) sin(z); -sin(z) cos(z)]*[1;0];
end

== matlab function Combined_Experiment_Jan23_2020a_NoArm/Phase #5: Hold Home/Change BLUE Behavior/Hough Control/MATLAB Function4 ==
  data: Oy input; e_out output; e_in input
function e_out = fcn(Oy, e_in)

a = sign(Oy'*e_in);
e_out = -a*norm(e_in);

== matlab function Combined_Experiment_Jan23_2020a_NoArm/Simulate Plant Dynamics/RED and ARM Dynamics/RED Only/RED Dynamics/RED Dynamics Model/MATLAB Function ==
  data: control_inputs input; x_ddot output; model_param parameter
function x_ddot = RED_dynamics(control_inputs, model_param)

%#codegen
% Fully define the size of x_ddot() for code generation:
x_ddot     = zeros(3,1);

% Extract the servicer model parameters from the model_param vector defined
% in initialize.m:
m_RED    = model_param(1);
I_RED    = model_param(2);

% Extract the control inputs from the control_input vector:
Fx        = control_inputs(1);              % [N]
Fy        = control_inputs(2);              % [N]
Tz        = control_inputs(3);              % [N.m]

% Calculate the state acceleration vector:
x_ddot(1) = Fx/m_RED;                      % [m/s^2]
x_ddot(2) = Fy/m_RED;                      % [m/s^2]
x_ddot(3) = Tz/I_RED;                      % [rad/s^2]

end

== matlab function Combined_Experiment_Jan23_2020a_NoArm/From Torque Command RW/Change RED Behavior/Calculate Saturated RPM Signal/Calculate RW RPM Increment ==
  data: Tz_Sat input; dRPM_RW output
function dRPM_RW = Calc_RW_RPM(Tz_Sat)

dRPM_RW =  (Tz_Sat/0.007244720)*(60/2/pi)*0.1;

end

== matlab function Combined_Experiment_Jan23_2020a_NoArm/From Torque Command RW/Change RED Behavior/Wheel RPM to PWM/Check if RW is Ready ==
  data: Status input; EnableSig output; WheelRPM_In input; WheelRPM_Out output
function [EnableSig, WheelRPM_Out] = Check_Wheel_Status(Status, WheelRPM_In)

if Status == 0
    EnableSig    = 1;
    WheelRPM_Out = WheelRPM_In;
else
    EnableSig    = 0;
    WheelRPM_Out = 0;
end

end

== matlab function Combined_Experiment_Jan23_2020a_NoArm/From Torque Command RW/Change RED Behavior/Wheel RPM to PWM/Get RW Direction ==
  data: MotorRPM_Sat input; WheelDirection output
function WheelDirection = GetDirection(MotorRPM_Sat)

if MotorRPM_Sat > 0
    WheelDirection = 0;
else
    WheelDirection = 1;
end
        
end

== matlab function Combined_Experiment_Jan23_2020a_NoArm/From Torque Command RW/Change RED Behavior/Wheel RPM to PWM/RPM to PWM Value ==
  data: MotorRPM_Sat input; MotorPWM output
function MotorPWM = RPM2PWM(MotorRPM_Sat)

PWMRange = 0.9-0.1;

MotorPWM = ((MotorRPM_Sat*PWMRange)/7000) + 0.1;

end

== matlab function Combined_Experiment_Jan23_2020a_NoArm/Phase #3: Experiment/Change BLACK Behavior/Sub-Phase #3 /Hough Control/MATLAB Function4 ==
  data: Oy input; e_out output; e_in input
function e_out = fcn(Oy, e_in)

a = sign(Oy'*e_in);
e_out = -a*norm(e_in);

== matlab function Combined_Experiment_Jan23_2020a_NoArm/Phase #3: Experiment/Change BLACK Behavior/Sub-Phase #4/BLACK_RzD1/Wrap1/MATLAB Function ==
  data: u input; wrappedAngle output
function wrappedAngle = wrapAngle(u)

wrappedAngle = atan2(sin(u),cos(u));

end

== matlab function Combined_Experiment_Jan23_2020a_NoArm/Phase #3: Experiment/Change BLACK Behavior/Sub-Phase #4/Hough Control/MATLAB Function2 ==
  data: Oy output; z input; Ox output
function [Oy, Ox]   = C3( z )
%C3 gives the rotation matrix about the z-axis for an angle 'z'
%   z - the angle about the z-axis which you rotate
%   A - the rotation matrix

Ox = [cos(z) sin(z); -sin(z) cos(z)]*[1;0];
Oy = [cos(z) sin(z); -sin(z) cos(z)]*[0;1];
end

== matlab function Combined_Experiment_Jan23_2020a_NoArm/IMU Data and Algorithms/Change RED Behavior/Create Rotation Matrix ==
  data: Rz input; C_Ib output
function C_Ib = RotateFrame(Rz)

C_bI = [  cos(Rz) sin(Rz)
         -sin(Rz) cos(Rz) ];

C_Ib = inv(C_bI);

end

== matlab function Combined_Experiment_Jan23_2020a_NoArm/IMU Data and Algorithms/Change BLACK Behavior/Create Rotation Matrix ==
  data: Rz input; C_Ib output
function C_Ib = RotateFrame(Rz)

C_bI = [  cos(Rz) sin(Rz)
         -sin(Rz) cos(Rz) ];

C_Ib = inv(C_bI);

end

== matlab function Combined_Experiment_Jan23_2020a_NoArm/IMU Data and Algorithms/Change RED Behavior/ChangeOrientation ==
  data: u input; y output
function y = ChangeOrientation(u)

y = rotz(-90)*u';

== matlab function Combined_Experiment_Jan23_2020a_NoArm/IMU Data and Algorithms/Change BLACK Behavior/ChangeOrientation ==
  data: u input; y output
function y = ChangeOrientation(u)

y = rotz(-90)*u';

== matlab function Combined_Experiment_Jan23_2020a_NoArm/Simulate Plant Dynamics/BLACK Dynamics/BLACK Dynamics Model/MATLAB Function ==
  data: control_inputs input; x_ddot output; model_param parameter
function x_ddot = BLACK_dynamics(control_inputs, model_param)

%#codegen
% Fully define the size of x_ddot() for code generation:
x_ddot     = zeros(3,1);

% Extract the servicer model parameters from the model_param vector defined
% in initialize.m:
m_BLACK    = model_param(3);
I_BLACK    = model_param(4);

% Extract the control inputs from the control_input vector:
Fx        = control_inputs(1);              % [N]
Fy        = control_inputs(2);              % [N]
Tz        = control_inputs(3);              % [N.m]

% Calculate the state acceleration vector:
x_ddot(1) = Fx/m_BLACK;                      % [m/s^2]
x_ddot(2) = Fy/m_BLACK;                      % [m/s^2]
x_ddot(3) = Tz/I_BLACK;                      % [rad/s^2]

end

== matlab function Combined_Experiment_Jan23_2020a_NoArm/IMU Data and Algorithms/Change BLUE Behavior/ChangeOrientation ==
  data: u input; y output
function y = ChangeOrientation(u)

y = rotz(-90)*u';

== matlab function Combined_Experiment_Jan23_2020a_NoArm/IMU Data and Algorithms/Change BLUE Behavior/Create Rotation Matrix ==
  data: Rz input; C_Ib output
function C_Ib = RotateFrame(Rz)

C_bI = [  cos(Rz) sin(Rz)
         -sin(Rz) cos(Rz) ];

C_Ib = inv(C_bI);

end

== matlab function Combined_Experiment_Jan23_2020a_NoArm/Phase #3: Experiment/Change BLACK Behavior/Sub-Phase #4/Hough Control/MATLAB Function3 ==
  data: z input; Ox output
function Ox    = C3( z )
%C3 gives the rotation matrix about the z-axis for an angle 'z'
%   z - the angle about the z-axis which you rotate
%   A - the rotation matrix

Ox = [cos(z) sin(z); -sin(z) cos(z)]*[1;0];
end

== matlab function Combined_Experiment_Jan23_2020a_NoArm/Phase #3: Experiment/Change BLACK Behavior/Sub-Phase #4/Hough Control/MATLAB Function4 ==
  data: Oy input; e_out output; e_in input
function e_out = fcn(Oy, e_in)

a = sign(Oy'*e_in);
e_out = -a*norm(e_in);

== matlab function Combined_Experiment_Jan23_2020a_NoArm/Phase #3: Experiment/Change BLUE Behavior/Sub-Phase #1/Hough Control/MATLAB Function4 ==
  data: Oy input; e_out output; e_in input
function e_out = fcn(Oy, e_in)

a = sign(Oy'*e_in);
e_out = -a*norm(e_in);

== matlab function Combined_Experiment_Jan23_2020a_NoArm/Phase #3: Experiment/Change BLUE Behavior/Sub-Phase #2 /Hough Control/MATLAB Function4 ==
  data: Oy input; e_out output; e_in input
function e_out = fcn(Oy, e_in)

a = sign(Oy'*e_in);
e_out = -a*norm(e_in);

== matlab function Combined_Experiment_Jan23_2020a_NoArm/Phase #3: Experiment/Change BLUE Behavior/Sub-Phase #3 /BLACK_RzD1/Wrap1/MATLAB Function ==
  data: u input; wrappedAngle output
function wrappedAngle = wrapAngle(u)

wrappedAngle = atan2(sin(u),cos(u));

end
